simulink model "PD_simulinkfor1DOF"  (R2018a)
settings: Solver=VariableStepAuto  StartTime=0.0  StopTime=40  RelTol=1e-3
values from neighbouring files (symbols this model uses):
  B = 0.10    (= 0.1)    [initilize_parametersfor1DOF.m]
  g = 9.81    [initilize_parametersfor1DOF.m]
  I = 0.062    [initilize_parametersfor1DOF.m]
  L = 0.46    [initilize_parametersfor1DOF.m]
  Lc = 0.29    [initilize_parametersfor1DOF.m]
  m = 0.18    [initilize_parametersfor1DOF.m]
  M = 1.1    [initilize_parametersfor1DOF.m]
settings Model: Creator=Hung Dung  LastModifiedBy=Hung Dung
settings CodeAppCC: StateflowObjectComments=on

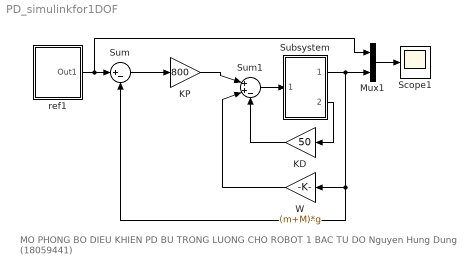
== system PD_simulinkfor1DOF ==
  note: MO PHONG BO DIEU KHIEN PD BU TRONG LUONG CHO ROBOT 1 BAC TU DO
      | Nguyen Hung Dung (18059441)
  KD : Gain  Gain=50
  KP : Gain  Gain=800
  Mux1 : Mux  Inputs=2
  Scope1 : Scope
  Subsystem : Subsystem
  Sum : Sum  Inputs=|+-
  Sum1 : Sum  Inputs=|++-
  W : Gain  Gain=(m+M)*g
  ref1 : Subsystem
  wires:
  Mux1/1 -> Scope1/1
  ref1/1(Out1) -> Mux1/1, Sum/1
  Sum1/1 -> Subsystem/1(U(t))
  Subsystem/1(Theta()) -> Sum/2, W/1, Mux1/2
  Subsystem/2(Theta()1) -> KD/1
  KD/1 -> Sum1/3
  W/1 -> Sum1/2
  KP/1 -> Sum1/1
  Sum/1 -> KP/1

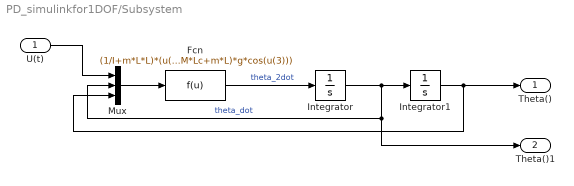
== system PD_simulinkfor1DOF/Subsystem ==
  U(t) : Inport
  Fcn : Fcn  Expr=(1/I+m*L*L)*(u(1)-B*u(2)-(M*Lc+m*L)*g*cos(u(3)))
  Integrator : Integrator  InitialCondition=pi/3
  Integrator1 : Integrator  InitialCondition=pi/3
  Mux : Mux  Inputs=3
  Theta() : Outport
  Theta()1 : Outport  Port=2
  wires:
  Fcn/1 -> Integrator/1  "theta_2dot"
  Integrator/1 -> Theta()1/1, Mux/2, Integrator1/1  "theta_dot"
  U(t)/1 -> Mux/1
  Mux/1 -> Fcn/1
  Integrator1/1 -> Theta()/1, Mux/3

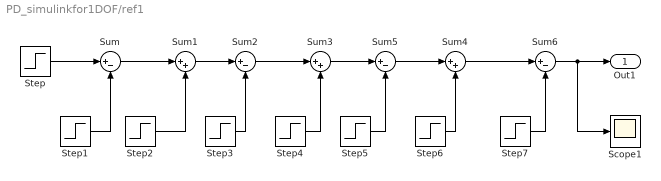
== system PD_simulinkfor1DOF/ref1 ==
  Scope1 : Scope
  Step : Step  Time=5  Before=pi/6  After=pi/6  SampleTime=0
  Step1 : Step  Time=5  After=pi/6  SampleTime=0
  Step2 : Step  Time=10  After=pi/3  SampleTime=0
  Step3 : Step  Time=15  After=pi/3  SampleTime=0
  Step4 : Step  Time=20  After=pi/2  SampleTime=0
  Step5 : Step  Time=25  After=pi/2  SampleTime=0
  Step6 : Step  Time=30  After=2*pi/3  SampleTime=0
  Step7 : Step  Time=35  After=2*pi/3  SampleTime=0
  Sum{,2,5..6} (4 alike) : Sum  Inputs=|+-  SaturateOnIntegerOverflow=on
  Sum1 : Sum  Inputs=|++  SaturateOnIntegerOverflow=on
  Sum3 : Sum  Inputs=|++  SaturateOnIntegerOverflow=on
  Sum4 : Sum  Inputs=|++  SaturateOnIntegerOverflow=on
  Out1 : Outport
  wires:
  Step/1 -> Sum/1
  Step1/1 -> Sum/2
  Sum/1 -> Sum1/1
  Step2/1 -> Sum1/2
  Sum1/1 -> Sum2/1
  Step3/1 -> Sum2/2
  Step4/1 -> Sum3/2
  Sum2/1 -> Sum3/1
  Sum3/1 -> Sum5/1
  Sum5/1 -> Sum4/1
  Step5/1 -> Sum5/2
  Step6/1 -> Sum4/2
  Sum4/1 -> Sum6/1
  Sum6/1 -> Scope1/1, Out1/1
  Step7/1 -> Sum6/2
